simulink model "Demo_M1V4_"  (R2018b)
settings: Solver=FixedStepDiscrete  StartTime=0.0  StopTime=inf  FixedStep=.03  RelTol=1e-3  EnableMultiTasking=on
libraries: MinSegLibrary_M1V4 x4, arduinolib x3, RASPlib x3
settings Model: SimulationMode=external  ExtModeTrigDuration=2  Creator=Alec  LastModifiedBy=j
settings DataIOCC: LimitDataPoints=on  SaveFormat=Array
settings OptimizationCC: EnhancedBackFolding=on  PassReuseOutputArgsAs=Individual arguments  ExpressionDepthLimit=2147483647  MaxStackSize=64  OptimizeBlockOrder=speed  DifferentSizesBufferReuse=on  OptimizationCustomize=off
settings DebuggingCC: UnderspecifiedInitializationDetection=Classic  MergeDetectMultiDrivingBlocksExec=none  ParameterTunabilityLossMsg=error  StateNameClashWarn=warning  SFUnexpectedBacktrackingDiag=warning  SFNoUnconditionalDefaultTransitionDiag=warning  SFExecutionAtInitializationDiag=none
settings HardwareCC: ProdBitPerInt=16  ProdBitPerPointer=16  ProdBitPerSizeT=16  ProdBitPerPtrDiffT=16  ProdLargestAtomicFloat=None  ProdWordSize=8  ProdHWDeviceType=Atmel->AVR  UseEmbeddedCoderFeatures=off  UseSimulinkCoderFeatures=off
settings ModelReferenceCC: PropagateSignalLabelsOutOfModel=off
settings SFSimCC: SimUseLocalCustomCode=off  MATLABDynamicMemAlloc=off
settings RTWCC: SystemTargetFile=ert.tlc  HardwareBoard=Arduino Mega 2560  TemplateMakefile=ert_default_tmf  GenerateReport=on  RTWVerbose=off  RTWUseLocalCustomCode=off  Toolchain=Arduino AVR  BuildConfiguration=Faster Runs  IncludeHyperlinkInReport=on  LaunchReport=on  GenerateTraceInfo=on  GenerateTraceReport=on  GenerateTraceReportSl=on  GenerateTraceReportSf=on  GenerateTraceReportEml=on
settings CodeAppCC: ForceParamTrailComments=on  IgnoreCustomStorageClasses=off  OperatorAnnotations=on  SimulinkDataObjDesc=on  SFDataObjDesc=on  MangleLength=10  CustomSymbolStrType=$N$R$M  InsertBlockDesc=on  InternalIdentifier=Classic
settings ERTTargetCC: SupportContinuousTime=on  SupportNonInlinedSFcns=on  SupportVariableSizeSignals=on
settings ConfigComp: CovMetricSettings=dw  CovHtmlReporting=on  CovSaveCumulativeToWorkspaceVar=on  CovSaveSingleToWorkspaceVar=on  CovExternalEMLEnable=off

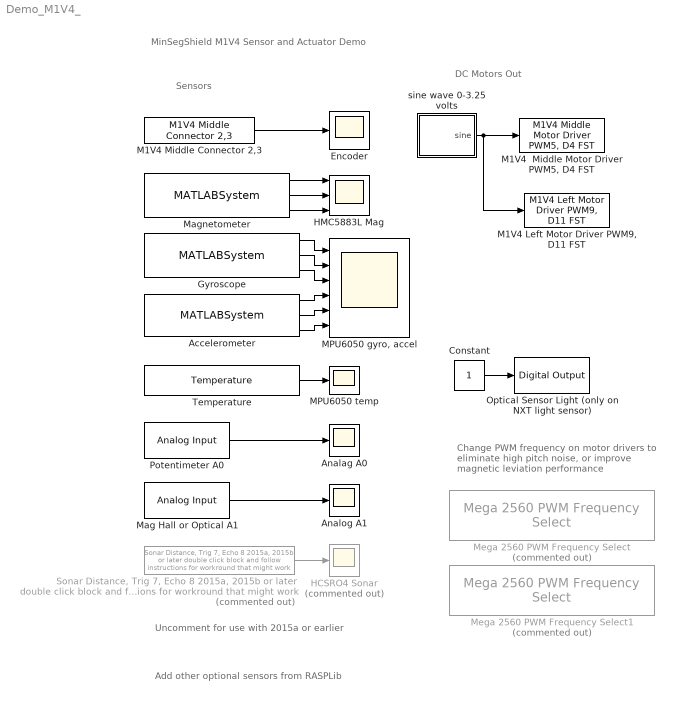
== system Demo_M1V4_ ==
  note: Add other optional sensors from RASPLib
  note: Uncomment for use with 2015a or earlier
  note: DC Motors Out
  note: Sensors
  note: MinSegShield M1V4 Sensor and Actuator Demo
  note: Change PWM frequency on motor drivers
      | to eliminate high pitch noise, or improve
      | magnetic leviation performance
  Accelerometer : MATLABSystem  System=soMPU6050Accel  SimulateUsing=Code generation
      mask Type: soMPU6050Accel
      mask Display:
      | disp('soMPU6050Accel');
      | port_label('output',1,'xaccel');
      | port_label('output',2,'yaccel');
      | port_label('output',3,'zaccel');
  Analag A0 : Scope
  Analog A1 : Scope
  Constant : Constant
  Encoder : Scope
  Gyroscope : MATLABSystem  System=soMPU6050Gyro  DLPFmode=0
      mask Type: soMPU6050Gyro
      mask Display:
      | disp('soMPU6050Gyro');
      | port_label('output',1,'xvel');
      | port_label('output',2,'yvel');
      | port_label('output',3,'zvel');
  HCSRO4 Sonar : Scope  Commented=on
  HMC5883L Mag : Scope  NumInputPorts=3
  "M1V4  Middle Motor Driver PWM5, D4 FST" : MinSegLibrary_M1V4/M1V4  Middle Motor Driver PWM5, D4 FST  Vsupply=3.25
      settings: SourceProductName=Rensselaer Arduino Support Package
  "M1V4 Left Motor Driver PWM9, D11 FST" : MinSegLibrary_M1V4/M1V4 Left Motor Driver PWM9, D11 FST  Vsupply=3.25
      settings: SourceProductName=Rensselaer Arduino Support Package
  M1V4 Middle Connector 2,3 : MinSegLibrary_M1V4/M1V4 Middle Connector 2,3  Encoder=0  PinA=3  PinB=2
      settings: SourceProductName=Rensselaer Arduino Support Package
  "MPU6050 gyro, accel" : Scope  NumInputPorts=6
  MPU6050 temp : Scope
  Mag Hall or Optical A1 : arduinolib/Analog Input  pinNumber=1  ReadResultsOnly=off  ConversionTriggerSource=Software  ExternalTriggerType=uint32(0)  OutputDataType=uint16  EnableConversionCompleteNotify=off  EnableOuputStatus=off  SampleTime=-1  blockPlatform=arduino
  Magnetometer : MATLABSystem  System=soHMC5883L  SimulateUsing=Code generation
      mask Type: soHMC5883L
      mask Display:
      | disp('soHMC5883L');
      | port_label('output',1,'xmag');
      | port_label('output',2,'ymag');
      | port_label('output',3,'zmag');
  Mega 2560 PWM Frequency Select : RASPlib/Mega 2560 PWM Frequency Select  Commented=on  Frequency=32KHz  Timer=2 - pins 9, 10
      settings: SourceProductName=Rensselaer Arduino Support Package
  Mega 2560 PWM Frequency Select1 : RASPlib/Mega 2560 PWM Frequency Select  Commented=on  Frequency=32KHz  Timer=3 - pins 2, 3, 5
      settings: SourceProductName=Rensselaer Arduino Support Package
  Optical Sensor Light (only on NXT light sensor) : arduinolib/Digital Output  pinNumber=12  blockPlatform=arduino
  Potentimeter A0 : arduinolib/Analog Input  pinNumber=0  ReadResultsOnly=off  ConversionTriggerSource=Software  ExternalTriggerType=uint32(0)  OutputDataType=uint16  EnableConversionCompleteNotify=off  EnableOuputStatus=off  SampleTime=-1  blockPlatform=arduino
  "Sonar Distance, Trig 7, Echo 8 2015a, 2015b or later double click block and follow instructions for workround that might work" : MinSegLibrary_M1V4/Sonar Distance, Trig 7, Echo 8 2015a, 2015b or later double click block and follow instructions for workround that might work  Commented=on  Sonar=1  TrigPin=7  EchoPin=8
      settings: SourceProductName=Rensselaer Arduino Support Package
  Temperature : RASPlib/Temperature  SimulateUsing=Code generation
      settings: SourceProductName=Rensselaer Arduino Support Package
  sine wave 0-3.25 volts : Subsystem
  wires:
  sine wave 0-3.25 volts/1(sine) -> "M1V4 Left Motor Driver PWM9, D11 FST"/1, "M1V4  Middle Motor Driver PWM5, D4 FST"/1
  Potentimeter A0/1 -> Analag A0/1
  Mag Hall or Optical A1/1 -> Analog A1/1
  Constant/1 -> Optical Sensor Light (only on NXT light sensor)/1
  M1V4 Middle Connector 2,3/1 -> Encoder/1
  "Sonar Distance, Trig 7, Echo 8 2015a, 2015b or later double click block and follow instructions for workround that might work"/1 -> HCSRO4 Sonar/1
  Gyroscope/1 -> "MPU6050 gyro, accel"/1
  Gyroscope/2 -> "MPU6050 gyro, accel"/2
  Gyroscope/3 -> "MPU6050 gyro, accel"/3
  Accelerometer/1 -> "MPU6050 gyro, accel"/4
  Accelerometer/2 -> "MPU6050 gyro, accel"/5
  Accelerometer/3 -> "MPU6050 gyro, accel"/6
  Magnetometer/1 -> HMC5883L Mag/1
  Magnetometer/2 -> HMC5883L Mag/2
  Magnetometer/3 -> HMC5883L Mag/3
  Temperature/1 -> MPU6050 temp/1

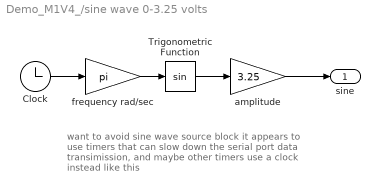
== system Demo_M1V4_/sine wave 0-3.25 volts ==
  note: want to avoid sine wave source block
      | it appears to use timers that can slow down the
      | serial port data transimission, and maybe
      | other timers
      |
      | use a clock instead like this
  Clock : Clock
  Trigonometric Function : Trigonometry
  amplitude : Gain  Gain=3.25
  frequency rad/sec : Gain  Gain=pi
  sine : Outport
  wires:
  Clock/1 -> frequency rad/sec/1
  Trigonometric Function/1 -> amplitude/1
  frequency rad/sec/1 -> Trigonometric Function/1
  amplitude/1 -> sine/1
